simulink model "Sim_0625"  (R2025b)
settings: Solver=ode4  StartTime=0.0  StopTime=3.14  FixedStep=0.001  RelTol=1e-3  EnableMultiTasking=on
settings Model: ExtModeTrigMode=oneshot  ExtModeArmWhenConnect=off  Creator=J  LastModifiedBy=J
settings DataIOCC: SaveFormat=Array  SignalLoggingSaveFormat=ModelDataLogs  ReturnWorkspaceOutputs=off  SignalLoggingName=sigsOut
settings OptimizationCC: BooleanDataType=off  ReuseModelBlockBuffer=off
settings DebuggingCC: SaveWithParameterizedLinksMsg=none  UnderspecifiedInitializationDetection=Classic  MergeDetectMultiDrivingBlocksExec=none  SignalResolutionControl=TryResolveAllWithWarning  MultiTaskDSMMsg=warning  MultiTaskCondExecSysMsg=none  UnconnectedInputMsg=warning  UnconnectedOutputMsg=warning  UnconnectedLineMsg=warning
settings HardwareCC: ProdBitPerPointer=32.0  ProdBitPerSizeT=32.0  ProdBitPerPtrDiffT=32.0  ProdLargestAtomicFloat=None  ProdIntDivRoundTo=Undefined  ProdEndianess=Unspecified  ProdWordSize=32.0  ProdHWDeviceType=32-bit Generic  TargetUnknown=on
settings ModelReferenceCC: PropagateSignalLabelsOutOfModel=off
settings RTWCC: GPUComputeCapability=3.5
settings GRTTargetCC: CombineOutputUpdateFcns=off  GRTInterface=on
settings ConfigComp: CovMetricSettings=dw  CovSaveCumulativeToWorkspaceVar=on  CovSaveSingleToWorkspaceVar=on
settings SimscapeCC: SimscapeLogDataHistory=5000  SimscapeLogDecimation=1

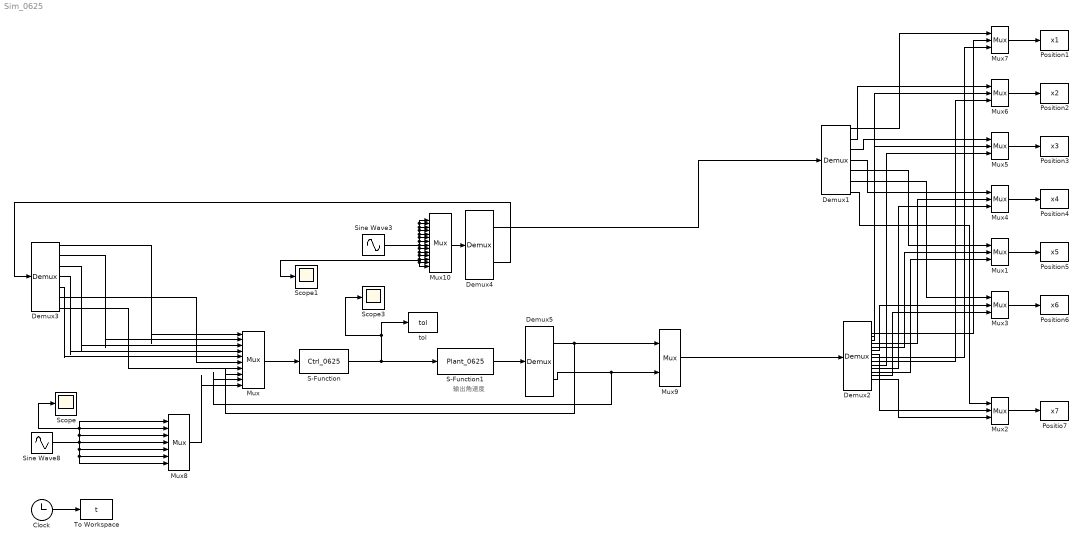
== system Sim_0625 ==
  note: 输出角速度
  Clock : Clock
  Demux1 : Demux  Outputs=7
      settings: DisplayOption=none
  Demux2 : Demux  Outputs=14
      settings: DisplayOption=none
  Demux3 : Demux  Outputs=7
      settings: DisplayOption=none
  Demux4 : Demux  Outputs=2
      settings: DisplayOption=none
  Demux5 : Demux  Outputs=2
      settings: DisplayOption=none
  Mux : Mux  Inputs=10
  Mux{1..7} (7 alike) : Mux  Inputs=3
  Mux10 : Mux  Inputs=14
  Mux8 : Mux  Inputs=7
  Mux9 : Mux  Inputs=2
  Positio7 : ToWorkspace  VariableName=x7  SampleTime=-1
  Position1 : ToWorkspace  VariableName=x1  SampleTime=-1
  Position2 : ToWorkspace  VariableName=x2  SampleTime=-1
  Position3 : ToWorkspace  VariableName=x3  SampleTime=-1
  Position4 : ToWorkspace  VariableName=x4  SampleTime=-1
  Position5 : ToWorkspace  VariableName=x5  SampleTime=-1
  Position6 : ToWorkspace  VariableName=x6  SampleTime=-1
  S-Function : S-Function  FunctionName=Ctrl_0625  SFunctionDeploymentMode=off  EnableBusSupport=off
  S-Function1 : S-Function  FunctionName=Plant_0625  SFunctionDeploymentMode=off  EnableBusSupport=off
  Scope : Scope
      settings: ActiveDisplayYMinimum=-3.06164647379911  ActiveDisplayYMaximum=2.8444089601561284
  Scope1 : Scope
      settings: ActiveDisplayYMinimum=-3.06164647379911  ActiveDisplayYMaximum=2.8444089601561284
  Scope3 : Scope
      settings: ActiveDisplayYMinimum=-33.260378228319453  ActiveDisplayYMaximum=38.151854111992932  DataLoggingVariableName=ScopeData3
  Sine Wave3 : Sin  Amplitude=0.3  Phase=pi/2  SampleTime=0
  Sine Wave8 : Sin  Amplitude=0.3  Phase=pi  SampleTime=0
  To Workspace : ToWorkspace  VariableName=t  SampleTime=-1
  tol : ToWorkspace  VariableName=tol  SampleTime=-1
  wires:
  Mux/1 -> S-Function/1
  Mux2/1 -> Positio7/1
  Mux3/1 -> Position6/1
  Clock/1 -> To Workspace/1
  Mux1/1 -> Position5/1
  Mux4/1 -> Position4/1
  Mux5/1 -> Position3/1
  Mux6/1 -> Position2/1
  Mux7/1 -> Position1/1
  Demux2/1 -> Mux7/2
  Demux2/2 -> Mux6/2
  Demux2/3 -> Mux5/2
  Demux2/4 -> Mux4/2
  Demux2/5 -> Mux1/2
  Demux2/6 -> Mux3/2
  Demux2/7 -> Mux2/2
  Demux2/8 -> Mux7/3
  Demux2/9 -> Mux6/3
  Demux2/10 -> Mux5/3
  Demux2/11 -> Mux4/3
  Demux2/12 -> Mux1/3
  Demux2/13 -> Mux3/3
  Demux2/14 -> Mux2/3
  S-Function/1 -> tol/1, Scope3/1, S-Function1/1
  Mux8/1 -> Mux/10
  Mux9/1 -> Demux2/1
  Demux4/1 -> Demux1/1
  Demux4/2 -> Demux3/1
  Demux3/1 -> Mux/1
  Demux3/2 -> Mux/2
  Demux3/3 -> Mux/3
  Demux3/4 -> Mux/4
  Demux3/5 -> Mux/5
  Demux3/6 -> Mux/6
  Demux3/7 -> Mux/7
  Demux1/1 -> Mux7/1
  Demux1/2 -> Mux6/1
  Demux1/3 -> Mux5/1
  Demux1/4 -> Mux4/1
  Demux1/5 -> Mux1/1
  Demux1/6 -> Mux3/1
  Demux1/7 -> Mux2/1
  Mux10/1 -> Demux4/1
  Sine Wave3/1 -> Mux10/1, Mux10/2, Mux10/3, Mux10/4, Mux10/5, Mux10/6, Mux10/7, Mux10/14, Mux10/13, Scope1/1, Mux10/12, Mux10/11, Mux10/10, Mux10/9, Mux10/8
  Sine Wave8/1 -> Mux8/7, Mux8/6, Mux8/5, Mux8/2, Scope/1, Mux8/1, Mux8/3, Mux8/4
  S-Function1/1 -> Demux5/1
  Demux5/1 -> Mux/8, Mux9/1
  Demux5/2 -> Mux/9, Mux9/2
